simulink model "3-3"  (R2022b)
settings: Solver=VariableStepAuto  StartTime=0.0  StopTime=10.0  RelTol=1e-3
settings Model: Creator=Mavara-(Asus)  LastModifiedBy=Mavara-(Asus)

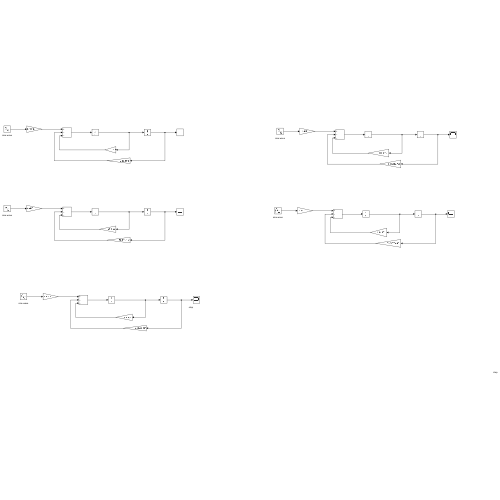
[thumbnail: Simulink's stored preview of the top-level diagram]
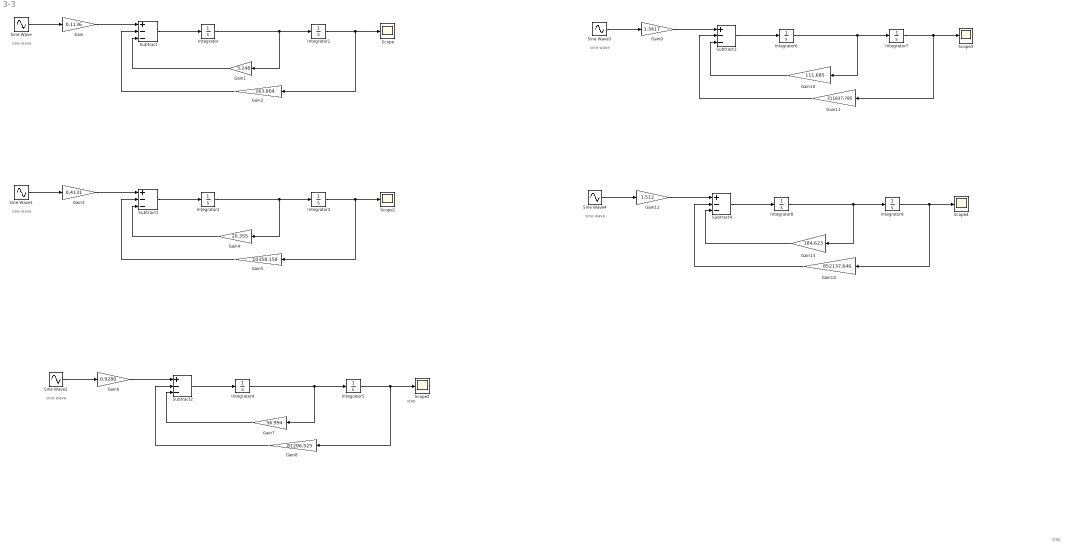
== system 3-3 ==
  note: sine wave
  note: step
  note: sine wave
  note: sine wave
  note: sine wave
  note: sine wave
  note: step
  Gain : Gain  Gain=0.1136
  Gain1 : Gain  Gain=3.248
  Gain10 : Gain  Gain=111.685
  Gain11 : Gain  Gain=311837.785
  Gain12 : Gain  Gain=1.512
  Gain13 : Gain  Gain=184.623
  Gain14 : Gain  Gain=852137.646
  Gain2 : Gain  Gain=263.804
  Gain3 : Gain  Gain=0.4131
  Gain4 : Gain  Gain=20.355
  Gain5 : Gain  Gain=10358.158
  Gain6 : Gain  Gain=0.9280
  Gain7 : Gain  Gain=56.994
  Gain8 : Gain  Gain=81206.525
  Gain9 : Gain  Gain=1.3417
  Integrator{,1..9} (10 alike) : Integrator
  Scope{,1..4} (5 alike) : Scope
  Sine Wave{,1..4} (5 alike) : Sin  SampleTime=0
  Subtract{,1..4} (5 alike) : Sum  Inputs=+--
  wires:
  Sine Wave/1 -> Gain/1
  Gain/1 -> Subtract/1
  Subtract/1 -> Integrator/1
  Integrator/1 -> Gain1/1, Integrator1/1
  Gain1/1 -> Subtract/3
  Gain2/1 -> Subtract/2
  Integrator1/1 -> Scope/1, Gain2/1
  Gain4/1 -> Subtract1/3
  Integrator2/1 -> Gain4/1, Integrator3/1
  Gain5/1 -> Subtract1/2
  Sine Wave1/1 -> Gain3/1
  Subtract1/1 -> Integrator2/1
  Gain3/1 -> Subtract1/1
  Integrator3/1 -> Scope1/1, Gain5/1
  Gain7/1 -> Subtract2/3
  Integrator4/1 -> Gain7/1, Integrator5/1
  Gain8/1 -> Subtract2/2
  Sine Wave2/1 -> Gain6/1
  Subtract2/1 -> Integrator4/1
  Gain6/1 -> Subtract2/1
  Integrator5/1 -> Scope2/1, Gain8/1
  Gain10/1 -> Subtract3/3
  Integrator6/1 -> Gain10/1, Integrator7/1
  Gain11/1 -> Subtract3/2
  Sine Wave3/1 -> Gain9/1
  Subtract3/1 -> Integrator6/1
  Gain9/1 -> Subtract3/1
  Integrator7/1 -> Scope3/1, Gain11/1
  Gain13/1 -> Subtract4/3
  Integrator8/1 -> Gain13/1, Integrator9/1
  Gain14/1 -> Subtract4/2
  Sine Wave4/1 -> Gain12/1
  Subtract4/1 -> Integrator8/1
  Gain12/1 -> Subtract4/1
  Integrator9/1 -> Scope4/1, Gain14/1
